simulink model "VCU_DriveControl"  (R2023b)
settings: Solver=FixedStepAuto  StartTime=0.0  StopTime=10.0  FixedStep=0.01  RelTol=1e-3
undefined symbols (not defined in the file or in its folder): DiscIntNeverNeededParam
libraries: simulink x10
settings Model: Creator=Administrator  LastModifiedBy=Administrator
settings OptimizationCC: DefaultParameterBehavior=Inlined  EnhancedBackFolding=on  PassReuseOutputArgsAs=Individual arguments  ZeroExternalMemoryAtStartup=off  ZeroInternalMemoryAtStartup=off  OptimizeBlockOrder=speed  DifferentSizesBufferReuse=on  OptimizationCustomize=off  EfficientTunableParamExpr=on
settings DebuggingCC: ParameterTunabilityLossMsg=error
settings HardwareCC: ProdBitPerPointer=32  ProdBitPerSizeT=32  ProdBitPerPtrDiffT=32  ProdLargestAtomicInteger=Long  ProdLargestAtomicFloat=Double  ProdWordSize=32  ProdHWDeviceType=ARM Compatible->ARM Cortex-M
settings SFSimCC: MATLABDynamicMemAlloc=off
settings RTWCC: Description=Embedded Coder  SystemTargetFile=ert.tlc  GenCodeOnly=on  TemplateMakefile=ert_default_tmf  GenerateReport=on  IncludeHyperlinkInReport=on  LaunchReport=on  GenerateTraceInfo=on  GenerateTraceReport=on  GenerateCodeReplacementReport=on
settings CodeAppCC: ForceParamTrailComments=on  IgnoreCustomStorageClasses=off  OperatorAnnotations=on  SimulinkDataObjDesc=on  SFDataObjDesc=on  InsertBlockDesc=on
settings ERTTargetCC: TargetLangStandard=C99 (ISO)  GenerateSampleERTMain=on  InlinedParameterPlacement=NonHierarchical  ERTCustomFileTemplate=example_file_process.tlc

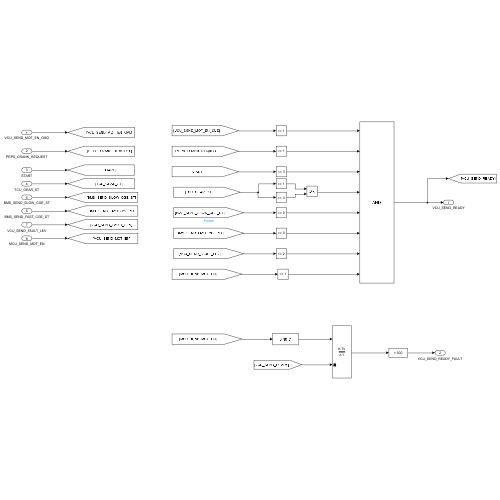
[thumbnail: Simulink's stored preview of the top-level diagram]
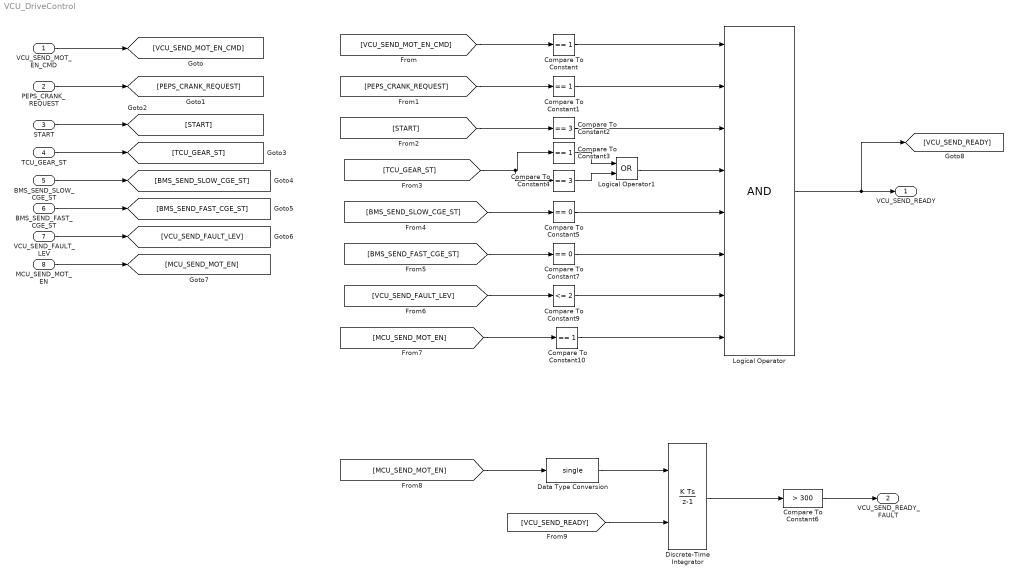
== system VCU_DriveControl ==
  VCU_SEND_MOT_EN_CMD : Inport
  PEPS_CRANK_REQUEST : Inport  Port=2
  START : Inport  Port=3
  TCU_GEAR_ST : Inport  Port=4
  BMS_SEND_SLOW_CGE_ST : Inport  Port=5
  BMS_SEND_FAST_CGE_ST : Inport  Port=6
  VCU_SEND_FAULT_LEV : Inport  Port=7
  MCU_SEND_MOT_EN : Inport  Port=8
  Compare To Constant{,1,3,10} (4 alike) : simulink/Logic and Bit Operations/Compare To Constant  relop===  const=1  OutDataTypeStr=boolean
  Compare To Constant2 : simulink/Logic and Bit Operations/Compare To Constant  relop===  const=3  OutDataTypeStr=boolean
  Compare To Constant4 : simulink/Logic and Bit Operations/Compare To Constant  relop===  const=3  OutDataTypeStr=boolean
  Compare To Constant5 : simulink/Logic and Bit Operations/Compare To Constant  relop===  const=0  OutDataTypeStr=boolean
  Compare To Constant6 : simulink/Logic and Bit Operations/Compare To Constant  relop=>  const=300  OutDataTypeStr=boolean
  Compare To Constant7 : simulink/Logic and Bit Operations/Compare To Constant  relop===  const=0  OutDataTypeStr=boolean
  Compare To Constant9 : simulink/Logic and Bit Operations/Compare To Constant  relop=<=  const=2  OutDataTypeStr=boolean
  Data Type Conversion : DataTypeConversion  OutDataTypeStr=single  SaturateOnIntegerOverflow=off  RndMeth=Floor
  Discrete-Time Integrator : DiscreteIntegrator  ExternalReset=sampled level  SampleTime=-1  ICPrevOutput=DiscIntNeverNeededParam  ICPrevScaledInput=DiscIntNeverNeededParam
  Logical Operator : Logic  Inputs=8  AllPortsSameDT=off  OutDataTypeStr=boolean
  Logical Operator1 : Logic  Operator=OR  AllPortsSameDT=off  OutDataTypeStr=boolean
  VCU_SEND_READY : Outport
  VCU_SEND_READY_FAULT : Outport  Port=2
  wires:
  VCU_SEND_MOT_EN_CMD/1 -> [VCU_SEND_MOT_EN_CMD]
  PEPS_CRANK_REQUEST/1 -> [PEPS_CRANK_REQUEST]
  START/1 -> [START]
  TCU_GEAR_ST/1 -> [TCU_GEAR_ST]
  BMS_SEND_SLOW_CGE_ST/1 -> [BMS_SEND_SLOW_CGE_ST]
  BMS_SEND_FAST_CGE_ST/1 -> [BMS_SEND_FAST_CGE_ST]
  VCU_SEND_FAULT_LEV/1 -> [VCU_SEND_FAULT_LEV]
  MCU_SEND_MOT_EN/1 -> [MCU_SEND_MOT_EN]
  [VCU_SEND_MOT_EN_CMD] -> Compare To Constant/1
  [PEPS_CRANK_REQUEST] -> Compare To Constant1/1
  [START] -> Compare To Constant2/1
  [TCU_GEAR_ST] -> Compare To Constant4/1, Compare To Constant3/1
  [BMS_SEND_SLOW_CGE_ST] -> Compare To Constant5/1
  Compare To Constant3/1 -> Logical Operator1/1
  Compare To Constant4/1 -> Logical Operator1/2
  [BMS_SEND_FAST_CGE_ST] -> Compare To Constant7/1
  [VCU_SEND_FAULT_LEV] -> Compare To Constant9/1
  [MCU_SEND_MOT_EN] -> Compare To Constant10/1
  Logical Operator1/1 -> Logical Operator/4
  Compare To Constant9/1 -> Logical Operator/7
  Compare To Constant10/1 -> Logical Operator/8
  Compare To Constant5/1 -> Logical Operator/5
  Compare To Constant7/1 -> Logical Operator/6
  Compare To Constant/1 -> Logical Operator/1
  Compare To Constant1/1 -> Logical Operator/2
  Compare To Constant2/1 -> Logical Operator/3
  Logical Operator/1 -> [VCU_SEND_READY], VCU_SEND_READY/1
  [MCU_SEND_MOT_EN] -> Data Type Conversion/1
  Data Type Conversion/1 -> Discrete-Time Integrator/1
  [VCU_SEND_READY] -> Discrete-Time Integrator/2
  Discrete-Time Integrator/1 -> Compare To Constant6/1
  Compare To Constant6/1 -> VCU_SEND_READY_FAULT/1
